simulink model "Oscilation"  (R2024b)
settings: Solver=FixedStepAuto  StartTime=0  StopTime=10.0  FixedStep=1e-3  RelTol=1e-3
settings Model: Creator=ROG  LastModifiedBy=ROG

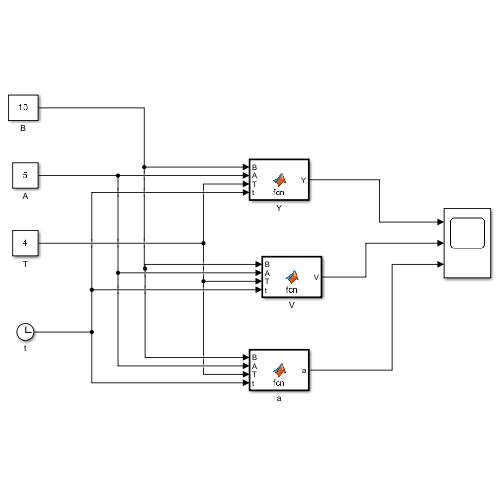
[thumbnail: Simulink's stored preview of the top-level diagram]
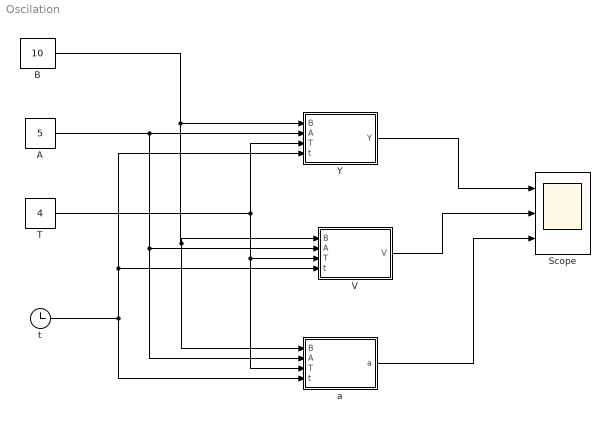
== system Oscilation ==
  A : Constant  Value=5
  B : Constant  Value=10
  Scope : Scope  NumInputPorts=3
  T : Constant  Value=4
  V : MATLAB Function  TreatAsAtomicUnit=on
  Y : MATLAB Function  TreatAsAtomicUnit=on
  a : MATLAB Function  TreatAsAtomicUnit=on
  t : Clock
      settings: Decimation=18
  wires:
  Y/1(Y) -> Scope/1
  V/1(V) -> Scope/2
  a/1(a) -> Scope/3
  B/1 -> Y/1(B), a/1(B), V/1(B)
  A/1 -> a/2(A), V/2(A), Y/2(A)
  T/1 -> a/3(T), V/3(T), Y/3(T)
  t/1 -> V/4(t), Y/4(t), a/4(t)

== matlab function Oscilation/V ==
  data: B input; V output; A input; T input; t input
function V= fcn(B,A,T,t)

V = 2*pi/T*A*cos(2*pi/T*t);

== matlab function Oscilation/Y ==
  data: B input; Y output; A input; T input; t input
function Y = fcn(B,A,T,t)

Y = B+A*sin(2*pi/T*t);

== matlab function Oscilation/a ==
  data: B input; a output; A input; T input; t input
function  a= fcn(B,A,T,t)

a = 2*pi/T*2*pi/T*A*-1*sin(2*pi/T*t);
